simulink model "closed_loop_model"  (R2023b)
settings: Solver=VariableStepAuto  StartTime=0.0  StopTime=0.83327  RelTol=1e-3
InitFcn:
  | load('SimulinkParams.mat');
values from neighbouring files (symbols this model uses):
  maxLag = M.maxLag    [SimulinkDataPrep.m]    (also in multi_data_MLP.m = max([significant_input_lags(:); top_output_lags(:)]); simulink_predict.m = 0)
  muX = muX(:)    [SimulinkDataPrep.m]
  muY = M.muY    [SimulinkDataPrep.m]
  sigmaX = sigmaX(:)    [SimulinkDataPrep.m]
  sigmaY = M.sigmaY    [SimulinkDataPrep.m]
  significant_input_lags = lags_cc_pos_ref(cc_mean > confidence_threshold)    [NARX_Input_ID_Time_Series_Methods.m]    (also in SimulinkDataPrep.m = M.significant_input_lags)
  top_output_lags = top_output_lags_sorted(keep)    [NARX_Input_ID_Time_Series_Methods.m]    (also in SimulinkDataPrep.m = M.top_output_lags)
libraries: cstblocks x2, deeplib x1
settings Model: Creator=MUSTAFAUGUR  LastModifiedBy=MUSTAFAUGUR

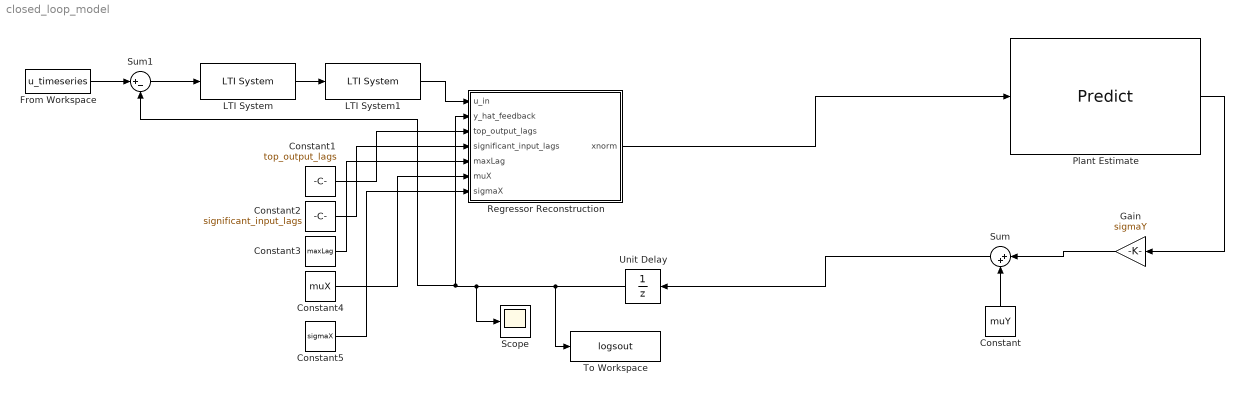
== system closed_loop_model ==
  Constant : Constant  Value=muY
  Constant1 : Constant  Value=top_output_lags
  Constant2 : Constant  Value=significant_input_lags
  Constant3 : Constant  Value=maxLag
  Constant4 : Constant  Value=muX
  Constant5 : Constant  Value=sigmaX
  From Workspace : FromWorkspace  VariableName=u_timeseries
  Gain : Gain  Gain=sigmaY
  LTI System : cstblocks/LTI System  sys=C_optd  IC=[]  PadeOrder=0
  LTI System1 : cstblocks/LTI System  sys=notchD  IC=[]  PadeOrder=0
  Plant Estimate : deeplib/Predict  Network=Network from MAT-file  NetworkFunction=squeezenet  NetworkFilePath=C:\Users\MUSTAFAUGUR\Desktop\ArdaGencer\MLP_model.mat  MiniBatchSize=128  InputDataFormats={'',''}  Predictions=on  Activations={}  ForceInterpretedSim=off  EnableDLNetwork=on
  Regressor Reconstruction : MATLAB Function  TreatAsAtomicUnit=on
  Scope : Scope
  Sum : Sum  Inputs=|++
  Sum1 : Sum  Inputs=|+-
  To Workspace : ToWorkspace  VariableName=logsout  SaveFormat=Timeseries  SampleTime=-1
  Unit Delay : UnitDelay  SampleTime=-1  HasFrameUpgradeWarning=on
  wires:
  Regressor Reconstruction/1(xnorm) -> Plant Estimate/1
  LTI System/1 -> LTI System1/1
  LTI System1/1 -> Regressor Reconstruction/1(u_in)
  Unit Delay/1 -> To Workspace/1, Scope/1, Sum1/2, Regressor Reconstruction/2(y_hat_feedback)
  Plant Estimate/1 -> Gain/1
  Gain/1 -> Sum/1
  Constant/1 -> Sum/2
  Sum/1 -> Unit Delay/1
  From Workspace/1 -> Sum1/1
  Sum1/1 -> LTI System/1
  Constant1/1 -> Regressor Reconstruction/3(top_output_lags)
  Constant2/1 -> Regressor Reconstruction/4(significant_input_lags)
  Constant3/1 -> Regressor Reconstruction/5(maxLag)
  Constant4/1 -> Regressor Reconstruction/6(muX)
  Constant5/1 -> Regressor Reconstruction/7(sigmaX)

== matlab function closed_loop_model/Regressor Reconstruction ==
  data: u_in input; xnorm output; y_hat_feedback input; top_output_lags input; significant_input_lags input; maxLag input; muX input; sigmaX input
function xnorm = buildRegressorClosedLoop(u_in, y_hat_feedback, top_output_lags, significant_input_lags, maxLag, muX, sigmaX)
%#codegen
persistent yBuf uBuf initialized

if isempty(initialized)
    yBuf = zeros(maxLag, 1);
    uBuf = zeros(maxLag+1, 1);
    initialized = true;
end

yBuf = [yBuf(2:end); y_hat_feedback];
uBuf = [uBuf(2:end); u_in];

yReg = yBuf(maxLag - top_output_lags + 1);
uReg = uBuf(maxLag+1 - significant_input_lags);

x = [yReg(:); uReg(:)];
xnorm = ((x - muX(:)) ./ sigmaX(:))';   % transpose to 1 x 55 row vector

end
